simulink model "MATLAB_Exercise_9question1to3"  (R2017b)
settings: Solver=FixedStepAuto  StartTime=0.0  StopTime=10  FixedStep=0.0001  RelTol=1e-3
libraries: simulink x2
settings Model: Creator=chenjiasheng  LastModifiedBy=chenjiasheng

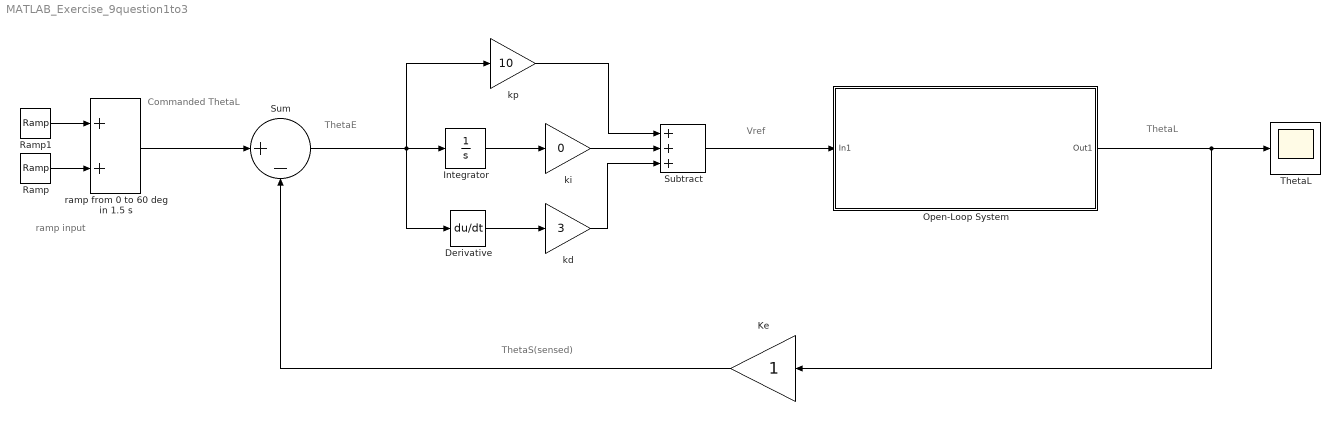
== system MATLAB_Exercise_9question1to3 ==
  note: ramp input
  note: Vref
  note: ThetaE
  note: ThetaS(sensed)
  note: ThetaL
  note: Commanded
      | ThetaL
  Derivative : Derivative
  Integrator : Integrator
  Ke : Gain
  Open-Loop System : Subsystem
  Ramp : simulink/Sources/Ramp  slope=40  start=0  X0=0
  Ramp1 : simulink/Sources/Ramp  slope=-40  start=1.5  X0=0
  Subtract : Sum  Inputs=+++
  Sum : Sum  Inputs=|+-
  ThetaL : Scope
  kd : Gain  Gain=3
  ki : Gain  Gain=0
  kp : Gain  Gain=10
  ramp from 0 to 60 deg in 1.5 s : Sum
  wires:
  Open-Loop System/1(Out1) -> Ke/1, ThetaL/1
  Sum/1 -> Derivative/1, Integrator/1, kp/1
  kp/1 -> Subtract/1
  Subtract/1 -> Open-Loop System/1(In1)
  Ke/1 -> Sum/2
  Integrator/1 -> ki/1
  ki/1 -> Subtract/2
  kd/1 -> Subtract/3
  Derivative/1 -> kd/1
  Ramp1/1 -> ramp from 0 to 60 deg in 1.5 s/1
  Ramp/1 -> ramp from 0 to 60 deg in 1.5 s/2
  ramp from 0 to 60 deg in 1.5 s/1 -> Sum/1

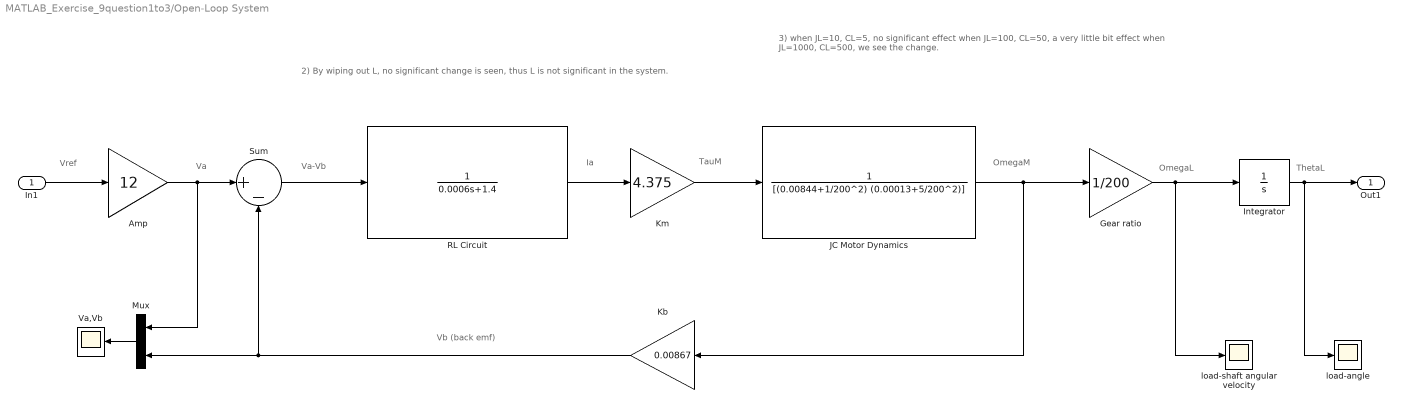
== system MATLAB_Exercise_9question1to3/Open-Loop System ==
  note: 3) when JL=10, CL=5, no significant effect
      | when JL=100, CL=50, a very little bit effect
      | when JL=1000, CL=500, we see the change.
  note: 2) By wiping out L, no significant change is seen, thus L is not significant in the system.
  note: OmegaL
  note: OmegaM
  note: TauM
  note: Ia
  note: Va-Vb
  note: Va
  note: Vb (back emf)
  note: Vref
  note: ThetaL
  In1 : Inport
  " load-shaft angular velocity" : Scope
  Amp : Gain  Gain=12
  Gear ratio : Gain  Gain=1/200
  Integrator : Integrator
  JC Motor Dynamics : TransferFcn  Denominator=[(0.00844+1/200^2) (0.00013+5/200^2)]
  Kb : Gain  Gain=0.00867
  Km : Gain  Gain=4.375
  Mux : Mux  Inputs=2
  RL Circuit : TransferFcn  Denominator=[0.0006 1.4]
  Sum : Sum  Inputs=|+-
  Va,Vb : Scope
  load-angle : Scope
  Out1 : Outport
  wires:
  RL Circuit/1 -> Km/1
  Amp/1 -> Sum/1, Mux/1
  Sum/1 -> RL Circuit/1
  Km/1 -> JC Motor Dynamics/1
  JC Motor Dynamics/1 -> Kb/1, Gear ratio/1
  Kb/1 -> Mux/2, Sum/2
  Gear ratio/1 -> " load-shaft angular velocity"/1, Integrator/1
  In1/1 -> Amp/1
  Integrator/1 -> load-angle/1, Out1/1
  Mux/1 -> Va,Vb/1
